simulink model "TestLibrary"  (R2018a)
settings: Solver=VariableStepAuto  StartTime=0.0  StopTime=1  RelTol=1e-3
libraries: TestLibrary_LIB x2
settings Model: Creator=Choaib ELMADI  LastModifiedBy=Choaib ELMADI

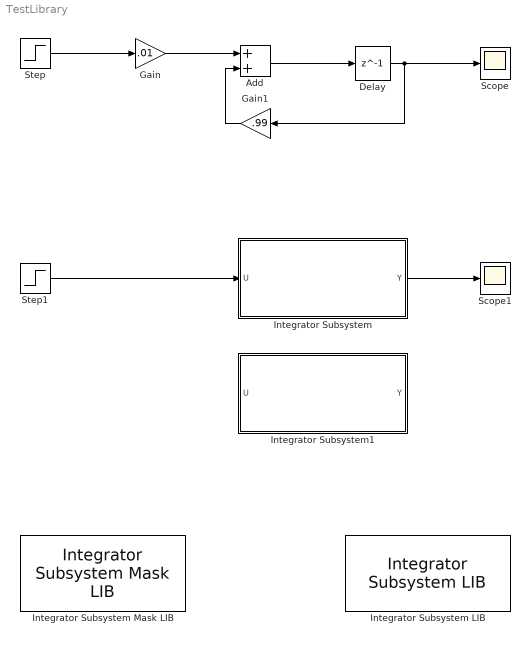
== system TestLibrary ==
  Add : Sum
  Delay : Delay  DelayLength=1
  Gain : Gain  Gain=.01
  Gain1 : Gain  Gain=.99
  Integrator Subsystem : Subsystem
  Integrator Subsystem LIB : TestLibrary_LIB/Integrator Subsystem LIB
  Integrator Subsystem Mask LIB : TestLibrary_LIB/Integrator Subsystem Mask LIB  FF=.02  FB=.97
  Integrator Subsystem1 : Subsystem  mask{FF=.03, FB=.97}
      mask prompts: FF "Feedforward Gain"; FB "Feedback Gain"
  Scope : Scope
  Scope1 : Scope
  Step : Step  Time=0  SampleTime=1e-3
  Step1 : Step  Time=0  SampleTime=1e-3
  wires:
  Add/1 -> Delay/1
  Gain/1 -> Add/1
  Delay/1 -> Scope/1, Gain1/1
  Gain1/1 -> Add/2
  Step/1 -> Gain/1
  Step1/1 -> Integrator Subsystem/1(U)
  Integrator Subsystem/1(Y) -> Scope1/1

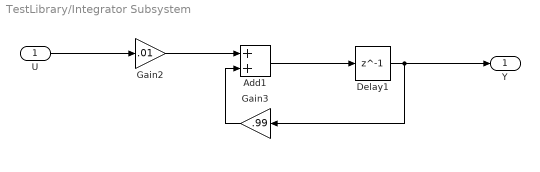
== system TestLibrary/Integrator Subsystem ==
  U : Inport
  Add1 : Sum
  Delay1 : Delay  DelayLength=1
  Gain2 : Gain  Gain=.01
  Gain3 : Gain  Gain=.99
  Y : Outport
  wires:
  Gain3/1 -> Add1/2
  Delay1/1 -> Y/1, Gain3/1
  Gain2/1 -> Add1/1
  Add1/1 -> Delay1/1
  U/1 -> Gain2/1

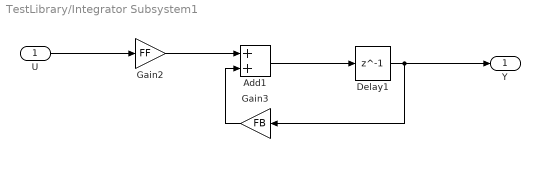
== system TestLibrary/Integrator Subsystem1 ==
  U : Inport
  Add1 : Sum
  Delay1 : Delay  DelayLength=1
  Gain2 : Gain  Gain=FF
  Gain3 : Gain  Gain=FB
  Y : Outport
  wires:
  U/1 -> Gain2/1
  Add1/1 -> Delay1/1
  Gain2/1 -> Add1/1
  Delay1/1 -> Gain3/1, Y/1
  Gain3/1 -> Add1/2
